simulink model "EE141ProjectSimulink"  (R2018a)
settings: Solver=VariableStepAuto  StartTime=0.0  StopTime=100  RelTol=1e-3
libraries: simulink x2
settings Model: Creator=michael  LastModifiedBy=michael

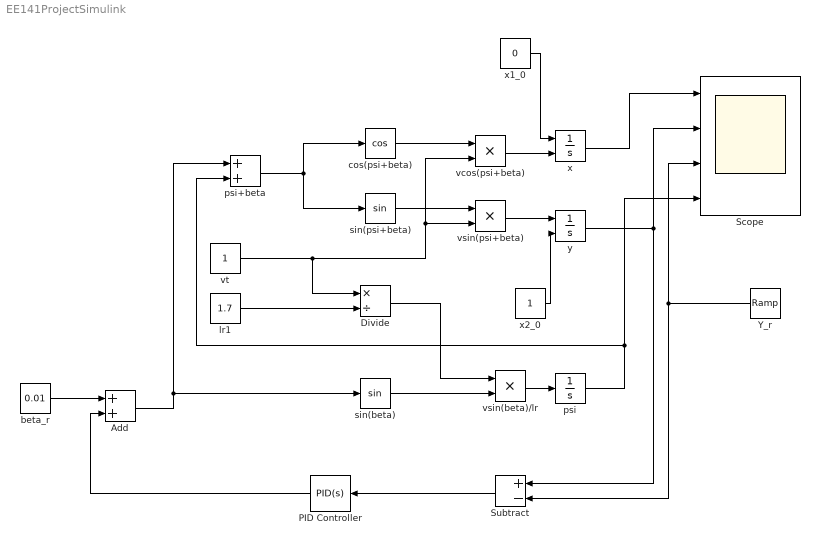
== system EE141ProjectSimulink ==
  Add : Sum
  Divide : Product  Inputs=*/
  PID Controller : simulink/Continuous/PID Controller  Controller=PID  TimeDomain=Continuous-time  SampleTime=-1  IntegratorMethod=Forward Euler  FilterMethod=Forward Euler  Form=Parallel  UseFilter=on  ControllerParametersSource=internal  P=0  I=0  D=1000  N=0  InitialConditionSource=internal  InitialConditionForIntegrator=0  InitialConditionForFilter=0  ExternalReset=none  LimitOutput=off  UpperSaturationLimit=inf  LowerSaturationLimit=-inf  LinearizeAsGain=on  AntiWindupMode=none  Kb=1  TrackingMode=off  Kt=1  PParamMin=[]  PParamMax=[]  IParamMin=[]  IParamMax=[]  DParamMin=[]  DParamMax=[]  NParamMin=[]  NParamMax=[]  KbParamMin=[]  KbParamMax=[]  KtParamMin=[]  KtParamMax=[]  POutMin=[]  POutMax=[]  IOutMin=[]  IOutMax=[]  DOutMin=[]  DOutMax=[]  NOutMin=[]  NOutMax=[]  KbOutMin=[]  KbOutMax=[]  KtOutMin=[]  KtOutMax=[]  IntegratorOutMin=[]  IntegratorOutMax=[]  FilterOutMin=[]  FilterOutMax=[]  SumOutMin=[]  SumOutMax=[]  SumI1OutMin=[]  SumI1OutMax=[]  SumI2OutMin=[]  SumI2OutMax=[]  SumI3OutMin=[]  SumI3OutMax=[]  SumDOutMin=[]  SumDOutMax=[]  SaturationOutMin=[]  SaturationOutMax=[]  IntegratorContinuousStateAttributes=''  IntegratorStateMustResolveToSignalObject=off  IntegratorRTWStateStorageClass=Auto  FilterContinuousStateAttributes=''  FilterStateMustResolveToSignalObject=off  FilterRTWStateStorageClass=Auto  DifferentiatorICPrevScaledInput=0  DifferentiatorOutMin=[]  DifferentiatorOutMax=[]  FilterDiffOutCoefMin=[]  FilterDiffOutCoefMax=[]  SumDenOutMin=[]  SumDenOutMax=[]  SumNumOutMin=[]  SumNumOutMax=[]  ReciprocalOutMin=[]  ReciprocalOutMax=[]  DivideOutMin=[]  DivideOutMax=[]  TunerSelectOption=Transfer Function Based (PID Tuner App)
  Scope : Scope  NumInputPorts=4
  Subtract : Sum  Inputs=+-
  Y_r : simulink/Sources/Ramp  slope=1  start=0  InitialOutput=0
  beta_r : Constant  Value=0.01
  cos(psi+beta) : Trigonometry  Operator=cos
  lr1 : Constant  Value=1.7
  psi : Integrator
  psi+beta : Sum
  sin(beta) : Trigonometry
  sin(psi+beta) : Trigonometry
  vcos(psi+beta) : Product
  vsin(beta)/lr : Product
  vsin(psi+beta) : Product
  vt : Constant
  x : Integrator  InitialConditionSource=external
  x1_0 : Constant  Value=0
  x2_0 : Constant
  y : Integrator  InitialConditionSource=external
  wires:
  beta_r/1 -> Add/1
  Add/1 -> psi+beta/1, sin(beta)/1
  psi+beta/1 -> sin(psi+beta)/1, cos(psi+beta)/1
  cos(psi+beta)/1 -> vcos(psi+beta)/1
  sin(psi+beta)/1 -> vsin(psi+beta)/1
  vt/1 -> vcos(psi+beta)/2, vsin(psi+beta)/2, Divide/1
  lr1/1 -> Divide/2
  Divide/1 -> vsin(beta)/lr/1
  sin(beta)/1 -> vsin(beta)/lr/2
  vcos(psi+beta)/1 -> x/2
  vsin(psi+beta)/1 -> y/1
  vsin(beta)/lr/1 -> psi/1
  psi/1 -> Scope/4, psi+beta/2
  x/1 -> Scope/1
  y/1 -> Scope/2, Subtract/1
  Y_r/1 -> Scope/3, Subtract/2
  Subtract/1 -> PID Controller/1
  PID Controller/1 -> Add/2
  x2_0/1 -> y/2
  x1_0/1 -> x/1
